simulink model "Simulation"  (R2020b)
settings: Solver=VariableStepAuto  StartTime=0.0  StopTime=4000  RelTol=1e-3
undefined symbols (not defined in the file): m, n
settings Model: Creator=Ryan  LastModifiedBy=zeron
settings DataIOCC: ReturnWorkspaceOutputs=off
settings DebuggingCC: ArithmeticOperatorsInVariantConditions=warning
settings SFSimCC: CustomCodeUndefinedFunction=UseInterfaceOnly

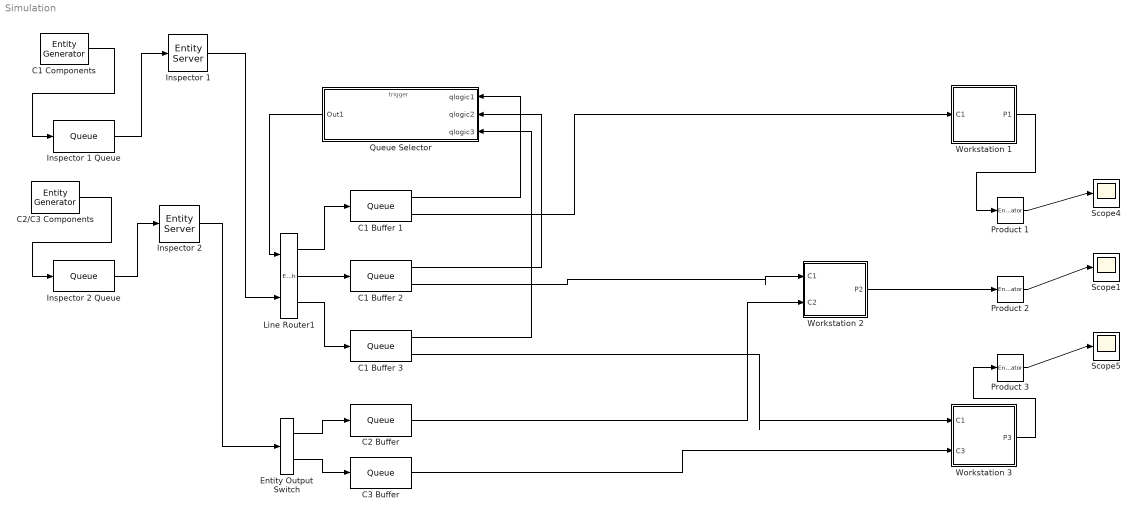
== system Simulation ==
  C1 Buffer 1 : Queue  InputPortMessageModes=m  OutputPortMessageModes=n,m  Capacity=2  NumberEntitiesInBlock=on
      settings: OutputPortMap=o1,o5
  C1 Buffer 2 : Queue  InputPortMessageModes=m  OutputPortMessageModes=n,m  Capacity=2  NumberEntitiesInBlock=on
      settings: OutputPortMap=o1,o5
  C1 Buffer 3 : Queue  InputPortMessageModes=m  OutputPortMessageModes=n,m  Capacity=2  NumberEntitiesInBlock=on
      settings: OutputPortMap=o1,o5
  C1 Components : EntityGenerator  OutputPortMessageModes=m  Period=0  AttributeName=entityType|outputPort  AttributeInitialValue=1|1  EntityType=Structured  EntityTypeName=Entity
  C2 Buffer : Queue  InputPortMessageModes=m  OutputPortMessageModes=m  Capacity=2
  C2/C3 Components : EntityGenerator  OutputPortMessageModes=m  Period=0  GenerateAction=|  AttributeName=entityType|outputPort  AttributeInitialValue=1|1  EntityType=Structured  EntityTypeName=Entity
      | % Generate a random entity type corresponding
      | % To the component type
      | entity.entityType = randi([2, 3])
      | 
      | % Define the output port
      | switch entity.entityType
      |     case 2
      |         entity.outputPort = 1
      |     case 3
      |         entity.outputPort = 2
      |     otherwise
      |         error('Invalid entity type')
      | end
  C3 Buffer : Queue  InputPortMessageModes=m  OutputPortMessageModes=m  Capacity=2
  Entity Output Switch : EntityOutputSwitch  InputPortMessageModes=m  OutputPortMessageModes=m,m  SwitchingCriterion=From attribute  SwitchAttributeName=outputPort
  Inspector 1 : EntityServer  InputPortMessageModes=m  OutputPortMessageModes=m  Capacity=1  ServiceTimeSource=MATLAB action  ServiceTimeAction=dt = wblrnd(10.725, 1.096);  EntryAction=|
      | % Entity will select the shortest queue
      | queuelogic();
  Inspector 1 Queue : Queue  InputPortMessageModes=m  OutputPortMessageModes=m
  "Inspector 2 " : EntityServer  InputPortMessageModes=m  OutputPortMessageModes=m  Capacity=1  ServiceTimeSource=MATLAB action  ServiceTimeAction=|
      | % Depending on the type of entity
      | % Generate the appropriate service time
      | switch entity.entityType
      |     case 2
      |         dt = wblrnd(16.0876, 1.09601);
      |     case 3
      |         dt = exprnd(20.6328);
      |     otherwise
      |         dt = -1
      | end
  Inspector 2 Queue : Queue  InputPortMessageModes=m  OutputPortMessageModes=m
  Line Router1 : EntityOutputSwitch  InputPortMessageModes=m,m  OutputPortMessageModes=m,m,m  NumberOutputPorts=3  SwitchingCriterion=From control port  SwitchAttributeName=QueuePath
      settings: InputPortMap=u0,u1  OutputPortMap=o0,o1,o2
  Product 1 : EntityTerminator  InputPortMessageModes=m  NumberEntitiesArrived=on
      settings: OutputPortMap=o0
  Product 2 : EntityTerminator  InputPortMessageModes=m  NumberEntitiesArrived=on
      settings: OutputPortMap=o0
  Product 3 : EntityTerminator  InputPortMessageModes=m  NumberEntitiesArrived=on
      settings: OutputPortMap=o0
  Queue Selector : Subsystem  TreatAsAtomicUnit=on
  Scope1 : Scope
  Scope4 : Scope
  Scope5 : Scope
  "Workstation 1 " : Subsystem
  Workstation 2 : Subsystem
  Workstation 3 : Subsystem
  wires:
  C1 Components/1 -> Inspector 1 Queue/1
  Inspector 1 Queue/1 -> Inspector 1/1
  C1 Buffer 1/1 -> Queue Selector/1(qlogic1)
  C1 Buffer 2/1 -> Queue Selector/2(qlogic2)
  C1 Buffer 3/1 -> Queue Selector/3(qlogic3)
  Inspector 1/1 -> Line Router1/2
  Queue Selector/1(Out1) -> Line Router1/1
  Line Router1/1 -> C1 Buffer 1/1
  Line Router1/2 -> C1 Buffer 2/1
  Line Router1/3 -> C1 Buffer 3/1
  C2/C3 Components/1 -> Inspector 2 Queue/1
  Inspector 2 Queue/1 -> "Inspector 2 "/1
  "Inspector 2 "/1 -> Entity Output Switch/1
  Entity Output Switch/1 -> C2 Buffer/1
  Entity Output Switch/2 -> C3 Buffer/1
  Product 1/1 -> Scope4/1
  C1 Buffer 1/2 -> "Workstation 1 "/1(C1)
  "Workstation 1 "/1(P1) -> Product 1/1
  C1 Buffer 2/2 -> Workstation 2/1(C1)
  C2 Buffer/1 -> Workstation 2/2(C2)
  Workstation 2/1(P2) -> Product 2/1
  C1 Buffer 3/2 -> Workstation 3/1(C1)
  C3 Buffer/1 -> Workstation 3/2(C3)
  Workstation 3/1(P3) -> Product 3/1
  Product 3/1 -> Scope5/1
  Product 2/1 -> Scope1/1

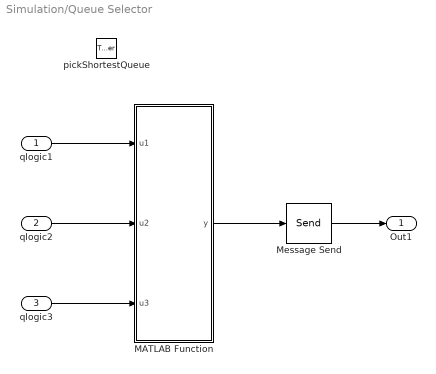
== system Simulation/Queue Selector ==
  qlogic1 : Inport
  qlogic2 : Inport  Port=2
  qlogic3 : Inport  Port=3
  pickShortestQueue : TriggerPort  TriggerType=function-call  IsSimulinkFunction=on  FunctionName=queuelogic  FunctionVisibility=scoped  VariantControl=Variant
  MATLAB Function : MATLAB Function  TreatAsAtomicUnit=on
  Message Send : Send  OutputPortMessageModes=m
  Out1 : Outport  VectorParamsAs1DForOutWhenUnconnected=off
  wires:
  qlogic1/1 -> MATLAB Function/1(u1)
  qlogic2/1 -> MATLAB Function/2(u2)
  qlogic3/1 -> MATLAB Function/3(u3)
  MATLAB Function/1(y) -> Message Send/1
  Message Send/1 -> Out1/1

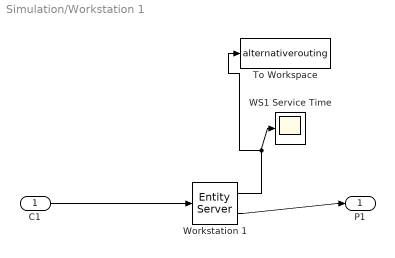
== system Simulation/Workstation 1  ==
  C1 : Inport
  To Workspace : ToWorkspace  VariableName=alternativerouting  SampleTime=-1
  WS1 Service Time : Scope
  Workstation 1 : EntityServer  InputPortMessageModes=m  OutputPortMessageModes=n,m  Capacity=1  ServiceTimeSource=MATLAB action  ServiceTimeValue=2  ServiceTimeAction=dt = exprnd(4.60442);  AverageWait=on
      settings: OutputPortMap=o4,o9
  P1 : Outport  VectorParamsAs1DForOutWhenUnconnected=off
  wires:
  Workstation 1/2 -> P1/1
  C1/1 -> Workstation 1/1
  Workstation 1/1 -> To Workspace/1, WS1 Service Time/1

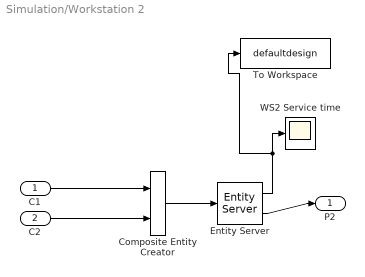
== system Simulation/Workstation 2 ==
  C1 : Inport
  C2 : Inport  Port=2
  Composite Entity Creator : CompositeEntityCreator  InputPortMessageModes=m,m  OutputPortMessageModes=m  EntityTypeName=Combined
      settings: InputPortMap=u0,u1
  Entity Server : EntityServer  InputPortMessageModes=m  OutputPortMessageModes=n,m  Capacity=1  ServiceTimeSource=MATLAB action  ServiceTimeValue=20  ServiceTimeAction=dt = wblrnd(10.6815, 0.922808);  AverageWait=on
      settings: OutputPortMap=o4,o9
  To Workspace : ToWorkspace  VariableName=defaultdesign  SampleTime=-1
  "WS2 Service time " : Scope
  P2 : Outport  VectorParamsAs1DForOutWhenUnconnected=off
  wires:
  C2/1 -> Composite Entity Creator/2
  Composite Entity Creator/1 -> Entity Server/1
  Entity Server/2 -> P2/1
  C1/1 -> Composite Entity Creator/1
  Entity Server/1 -> "WS2 Service time "/1, To Workspace/1

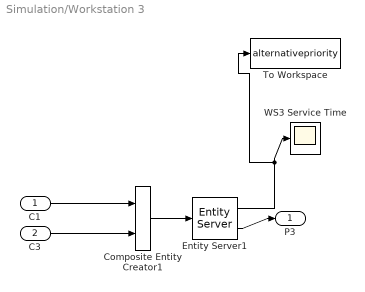
== system Simulation/Workstation 3 ==
  C1 : Inport
  C3 : Inport  Port=2
  Composite Entity Creator1 : CompositeEntityCreator  InputPortMessageModes=m,m  OutputPortMessageModes=m  EntityTypeName=Combined
      settings: InputPortMap=u0,u1
  Entity Server1 : EntityServer  InputPortMessageModes=m  OutputPortMessageModes=n,m  Capacity=1  ServiceTimeSource=MATLAB action  ServiceTimeValue=20  ServiceTimeAction=dt = exprnd(8.79558);  AverageWait=on
      settings: OutputPortMap=o4,o9
  To Workspace : ToWorkspace  VariableName=alternativepriority  SampleTime=-1
  WS3 Service Time : Scope
  P3 : Outport  VectorParamsAs1DForOutWhenUnconnected=off
  wires:
  Entity Server1/2 -> P3/1
  C3/1 -> Composite Entity Creator1/2
  Composite Entity Creator1/1 -> Entity Server1/1
  C1/1 -> Composite Entity Creator1/1
  Entity Server1/1 -> To Workspace/1, WS3 Service Time/1

== matlab function Simulation/Queue Selector/MATLAB Function ==
  data: u1 input; y output; u2 input; u3 input
function y = fcn(u1, u2, u3)
%#codegen

% Identify which input index is the smallest
[~,y] = min([u1 u2 u3]);
